simulink model "untitled"  (Simulink 8.4)
settings: Solver=ode45  StartTime=0.0  StopTime=10.0  FixedStep=0.001  RelTol=1e-3
settings Model: Creator=root
settings DataIOCC: SignalLoggingSaveFormat=Dataset
settings OptimizationCC: ExpressionDepthLimit=128
settings DebuggingCC: UnderspecifiedInitializationDetection=Simplified  MergeDetectMultiDrivingBlocksExec=error  FcnCallInpInsideContextMsg=EnableAllAsError  StateNameClashWarn=none
settings GRTTargetCC: CombineOutputUpdateFcns=on  GRTInterface=off

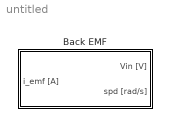
== system untitled ==
  Back EMF : Subsystem  TreatAsAtomicUnit=on

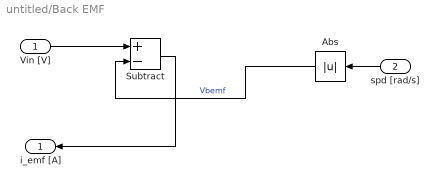
== system untitled/Back EMF ==
  Vin [V] : Inport
      settings: VarSizeSig=Yes
  spd [rad/s] : Inport  Port=2
  Abs : Abs
  Subtract : Sum  Inputs=+-
  i_emf [A] : Outport
  wires:
  Vin [V]/1 -> Subtract/1
  Subtract/1 -> i_emf [A]/1
  spd [rad/s]/1 -> Abs/1
  Abs/1 -> Subtract/2  "Vbemf"
